simulink model "rls2"  (Simulink 5.0)
settings: Solver=ode45  StartTime=0.0  StopTime=100.0  RelTol=1e-3
undefined symbols (not defined in the file): ts
libraries: dspmtrx3 x8, simulink x5, dspinverses x1
CloseFcn:
  | rtwprivate ssgensfun ModelCloseRequest rls
settings Model: LastModifiedBy=LeO

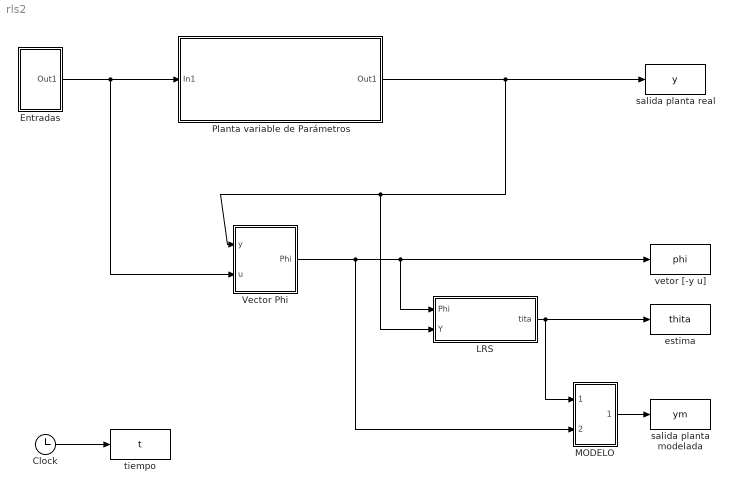
== system rls2 ==
  Clock : Clock
      settings: Decimation=10
  Entradas : Subsystem
  LRS : Subsystem
  MODELO : Subsystem
  Planta variable de Parámetros : Subsystem  mask{ruido=0.05, tiempo1=40}
      mask prompts: tiempo1 "tiempo de movimiento de parametros de la planta"
  Vector Phi : Subsystem  mask{nu=1, ny=3, nk=1}
      mask prompts: nu "Nº de u tomadas"; ny "Nº de y tomadas"; nk "Nº de retardo"
  estima : ToWorkspace  VariableName=thita  SampleTime=ts  SaveFormat=Array
  "salida planta modelada " : ToWorkspace  VariableName=ym  SampleTime=ts  SaveFormat=Array
  salida planta real : ToWorkspace  VariableName=y  SampleTime=ts  SaveFormat=Array
  "tiempo " : ToWorkspace  VariableName=t  SampleTime=ts  SaveFormat=Array
  vetor [-y u] : ToWorkspace  VariableName=phi  SampleTime=ts  SaveFormat=Array
  wires:
  Entradas/1(Out1) -> Planta variable de Parámetros/1(In1), Vector Phi/2(u)
  MODELO/1(Out1) -> "salida planta modelada "/1
  Clock/1 -> "tiempo "/1
  Planta variable de Parámetros/1(Out1) -> salida planta real/1, Vector Phi/1("y "), LRS/2(Y)
  LRS/1(tita) -> estima/1, MODELO/1(thita)
  Vector Phi/1(Phi) -> vetor [-y u]/1, LRS/1("Phi "), MODELO/2(Phi)

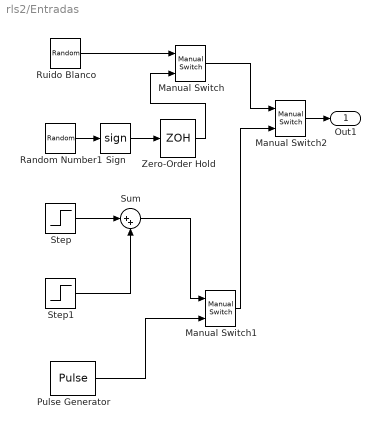
== system rls2/Entradas ==
  Manual Switch : simulink/Signal Routing/Manual Switch  sw=0  action=0
  Manual Switch1 : simulink/Signal Routing/Manual Switch  sw=1  action=0
  Manual Switch2 : simulink/Signal Routing/Manual Switch  sw=0  action=0
  Pulse Generator : DiscretePulseGenerator  PulseType=Time based  PulseWidth=50
  Random Number1 : RandomNumber  SampleTime=0
  Ruido Blanco : RandomNumber  Variance=20  Seed=12  SampleTime=ts
  Sign : Signum
  Step : Step  Time=10  After=25  SampleTime=0.05
  Step1 : Step  Time=50  After=5  SampleTime=0.05
  Sum : Sum  Inputs=|++  SaturateOnIntegerOverflow=on
  Zero-Order Hold : ZeroOrderHold  SampleTime=0.05
  Out1 : Outport
  wires:
  Sign/1 -> Zero-Order Hold/1
  Random Number1/1 -> Sign/1
  Manual Switch/1 -> Manual Switch2/1
  Ruido Blanco/1 -> Manual Switch/1
  Zero-Order Hold/1 -> Manual Switch/2
  Manual Switch2/1 -> Out1/1
  Step/1 -> Sum/1
  Step1/1 -> Sum/2
  Manual Switch1/1 -> Manual Switch2/2
  Sum/1 -> Manual Switch1/1
  Pulse Generator/1 -> Manual Switch1/2

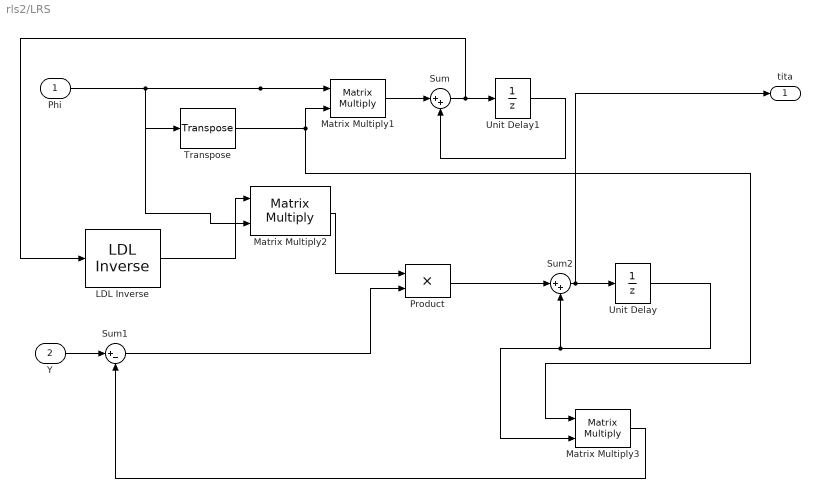
== system rls2/LRS ==
  "Phi " : Inport  SampleTime=ts
  Y : Inport  Port=2  SampleTime=ts
  LDL Inverse : dspinverses/LDL Inverse  errmode=Ignore
  Matrix Multiply1 : dspmtrx3/Matrix Multiply  numInputPorts=2  OptimizationLevel=None
  Matrix Multiply2 : dspmtrx3/Matrix Multiply  numInputPorts=2  OptimizationLevel=None
  Matrix Multiply3 : dspmtrx3/Matrix Multiply  numInputPorts=2  OptimizationLevel=None
  Product : Product  SaturateOnIntegerOverflow=on
  Sum : Sum  Inputs=|++  SaturateOnIntegerOverflow=on
  Sum1 : Sum  Inputs=|+-  SaturateOnIntegerOverflow=on
  Sum2 : Sum  Inputs=|++  SaturateOnIntegerOverflow=on
  Transpose : dspmtrx3/Transpose  Hermitian=off
  Unit Delay : UnitDelay  X0=1*10^-3  SampleTime=ts
  Unit Delay1 : UnitDelay  X0=10^-3  SampleTime=ts
  tita : Outport
  wires:
  "Phi "/1 -> Transpose/1, Matrix Multiply2/2, Matrix Multiply1/1
  Transpose/1 -> Matrix Multiply3/1, Matrix Multiply1/2
  Matrix Multiply1/1 -> Sum/1
  Sum/1 -> Unit Delay1/1, LDL Inverse/1
  Unit Delay1/1 -> Sum/2
  LDL Inverse/1 -> Matrix Multiply2/1
  Sum2/1 -> Unit Delay/1, tita/1
  Y/1 -> Sum1/1
  Matrix Multiply2/1 -> Product/1
  Product/1 -> Sum2/1
  Matrix Multiply3/1 -> Sum1/2
  Sum1/1 -> Product/2
  Unit Delay/1 -> Matrix Multiply3/2, Sum2/2

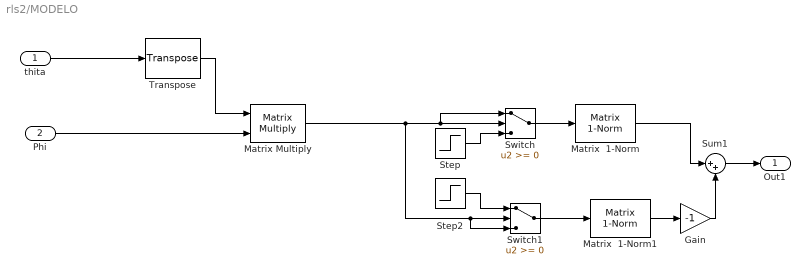
== system rls2/MODELO ==
  thita : Inport
  Phi : Inport  Port=2
  Gain : Gain  Gain=-1  SaturateOnIntegerOverflow=on
  Matrix  1-Norm : dspmtrx3/Matrix  1-Norm
  Matrix  1-Norm1 : dspmtrx3/Matrix  1-Norm
  Matrix Multiply : dspmtrx3/Matrix Multiply  numInputPorts=2  OptimizationLevel=None
  Step : Step  Time=0  After=0  SampleTime=0
  Step2 : Step  Time=0  After=0  SampleTime=0
  Sum1 : Sum  Inputs=|++  SaturateOnIntegerOverflow=on
  Switch : Switch  SaturateOnIntegerOverflow=on
  Switch1 : Switch  SaturateOnIntegerOverflow=on
  Transpose : dspmtrx3/Transpose  Hermitian=off
  Out1 : Outport
  wires:
  Phi/1 -> Matrix Multiply/2
  Transpose/1 -> Matrix Multiply/1
  thita/1 -> Transpose/1
  Matrix Multiply/1 -> Switch/2, Switch/1, Switch1/2, Switch1/3
  Sum1/1 -> Out1/1
  Step/1 -> Switch/3
  Switch/1 -> Matrix  1-Norm/1
  Switch1/1 -> Matrix  1-Norm1/1
  Step2/1 -> Switch1/1
  Matrix  1-Norm/1 -> Sum1/1
  Matrix  1-Norm1/1 -> Gain/1
  Gain/1 -> Sum1/2

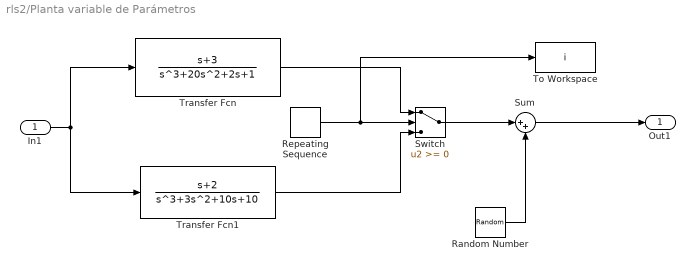
== system rls2/Planta variable de Parámetros ==
  In1 : Inport
  Random Number : RandomNumber  Variance=ruido  SampleTime=0
  Repeating Sequence : simulink/Sources/Repeating Sequence  rep_seq_t=[0 2*tiempo1]  rep_seq_y=[1 -1 ]
  Sum : Sum  Inputs=|++  SaturateOnIntegerOverflow=on
  Switch : Switch  SaturateOnIntegerOverflow=on
  To Workspace : ToWorkspace  VariableName=i  SampleTime=-1  SaveFormat=Array
  Transfer Fcn : TransferFcn  Numerator=[1 3 ]  Denominator=[1 20 2 1]
  Transfer Fcn1 : TransferFcn  Numerator=[1 2]  Denominator=[1 3 10 10]
  Out1 : Outport
  wires:
  Transfer Fcn/1 -> Switch/1
  Repeating Sequence/1 -> Switch/2, To Workspace/1
  Transfer Fcn1/1 -> Switch/3
  In1/1 -> Transfer Fcn/1, Transfer Fcn1/1
  Switch/1 -> Sum/1
  Sum/1 -> Out1/1
  Random Number/1 -> Sum/2

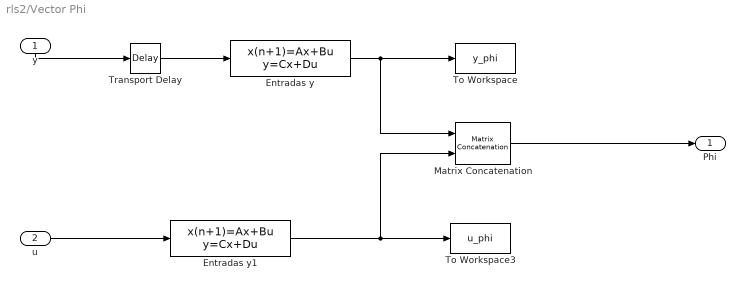
== system rls2/Vector Phi ==
  "y " : Inport  Orientation=down  SampleTime=ts
  u : Inport  Port=2  SampleTime=ts
  Entradas y : DiscreteStateSpace  A=[zeros(1,ny) ;eye(ny-1,ny)]  B=[[-1 zeros(1,ny-1)]']  C=[eye(ny)]  D=[zeros(1,ny)']  SampleTime=ts
  Entradas y1 : DiscreteStateSpace  A=[zeros(1,nu) ;eye(nu-1,nu)]  B=[[-1 zeros(1,nu-1)]']  C=[eye(nu)]  D=[zeros(1,nu)']  SampleTime=ts
  Matrix Concatenation : simulink/Math Operations/Matrix Concatenation  numInports=2  catMethod=Vertical
  To Workspace : ToWorkspace  VariableName=y_phi  SampleTime=ts  SaveFormat=Array
  To Workspace3 : ToWorkspace  VariableName=u_phi  SampleTime=ts  SaveFormat=Array
  Transport Delay : TransportDelay  DelayTime=nk*ts
  Phi : Outport
  wires:
  "y "/1 -> Transport Delay/1
  u/1 -> Entradas y1/1
  Entradas y/1 -> To Workspace/1, Matrix Concatenation/1
  Entradas y1/1 -> To Workspace3/1, Matrix Concatenation/2
  Matrix Concatenation/1 -> Phi/1
  Transport Delay/1 -> Entradas y/1
